simulink model "CombineAndExtractDataUsingVectors"  (R2013a)
settings: Solver=ode45  StartTime=0.0  StopTime=10.0  RelTol=1e-3
settings Model: Creator=ajdin  LastModifiedBy=ajdin

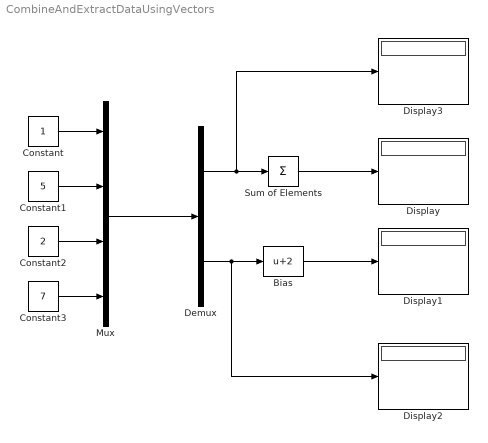
== system CombineAndExtractDataUsingVectors ==
  Bias : Bias  Bias=2
  Constant : Constant
  Constant1 : Constant  Value=5
  Constant2 : Constant  Value=2
  Constant3 : Constant  Value=7
  Demux : Demux  Outputs=2
  Display{,1..3} (4 alike) : Display
  Mux : Mux
  Sum of Elements : Sum  Inputs=+
  wires:
  Constant3/1 -> Mux/4
  Constant2/1 -> Mux/3
  Constant1/1 -> Mux/2
  Constant/1 -> Mux/1
  Mux/1 -> Demux/1
  Demux/2 -> Display2/1, Bias/1
  Demux/1 -> Display3/1, Sum of Elements/1
  Sum of Elements/1 -> Display/1
  Bias/1 -> Display1/1
